simulink model "SmartGrid"  (R2023a)
settings: Solver=FixedStepDiscrete  StartTime=0.0  StopTime=20  FixedStep=1e-6  RelTol=1e-3
undefined symbols (not defined in the file or in its folder): Ion, Lithium
libraries: spsSeriesRLCBranchLib x7, spsCurrentMeasurementLib x3, spsPWMGeneratorDCDCLib x3, spsMosfetLib x2, spsVoltageMeasurementLib x2, spsBatteryLib x1, spsPVArrayLib x1, spsDiodeLib x1, spsIGBTDiodeLib x1, spspowerguiLib x1
settings Model: Creator=Dishan Dey  LastModifiedBy=Dishan Dey

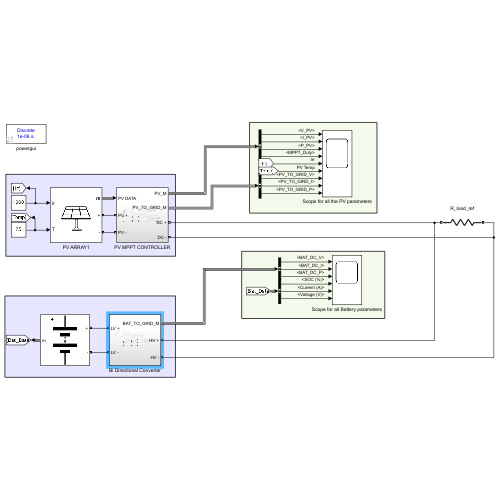
[thumbnail: Simulink's stored preview of the top-level diagram]
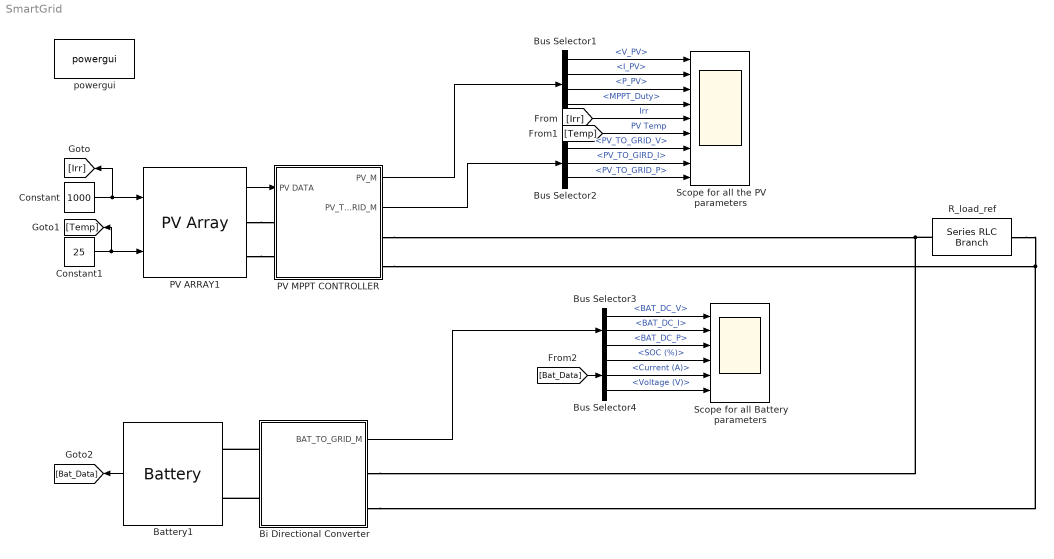
== system SmartGrid ==
  Battery1 : spsBatteryLib/Battery  BatType=Lithium-Ion  ShowTempParam=off  ThermalPreset=no  ShowAgeParam=off  NomV=48  NomQ=50  SOC=80  Batt_Tr=30  PresetModel=on  MaxQ=50  MinV=36  FullV=55.8714  Dis_rate=21.7391  R=0.0096  Normal_OP=45.2174  expZone="[51.8585      2.45652]"  current=[6.5 13 32.5]  Units=Time  Tci=20  NomT=20  T2=-30  MaxQ2=4.8  FullV2=7.1  Normal_OP2=5.655  expZone2="[6.58           1]"  Rca=0.6  ti=2000  Dp=0  Neq0=0  Tsim=1e6  Ta1=25  Qeol=5.4*0.9  Reol=0.013333*1.2  Char_age=[2.3478, 3]  Dis_age=[2.3478, 10]  N1=1500  N2=10500  N3=1000  N4=1400  Ta2=45  N5=950
  Bi Directional Converter : Subsystem
  Bus Selector1 : BusSelector  OutputSignals=V_PV,I_PV,P_PV,MPPT_Duty
  Bus Selector2 : BusSelector  OutputSignals=PV_TO_GRID_V,PV_TO_GIRD_I,PV_TO_GRID_P
  Bus Selector3 : BusSelector  OutputSignals=BAT_DC_V,BAT_DC_I,BAT_DC_P
  Bus Selector4 : BusSelector  OutputSignals=SOC (%),Current (A),Voltage (V)
  Constant : Constant  Value=1000  SampleTime=-1
  Constant1 : Constant  Value=25  SampleTime=-1
  PV ARRAY1 : spsPVArrayLib/PV Array  Npar=6  Nser=1  PlotType=array @ 25 deg.C & specified irradiances  S_vec="[ 1000  500  100 ]"  Temp_C_vec="[ 45 25  ]"  ModuleName=Canadian Solar Inc. CS6P-250P  PlotWhenSelected=off  Pm=249.83  Ncell=60  Voc=37.2  Isc=8.87  Vm=30.1  Im=8.3  beta_Voc_pc=-0.301  alpha_Isc_pc=0.038997  beta_Voc=-0.11197  alpha_Isc=0.003459  IL=8.8849  I0=3.0928e-11  nI=0.91537  Rsh=202.8148  Rs=0.34115  RobustModel=off  RobustCellTemperature=313.3991  BAL=on  Tc=1e-6  Tfilter=5e-5
  PV MPPT CONTROLLER : Subsystem
  R_load_ref : spsSeriesRLCBranchLib/Series RLC Branch  LConnTagsString=__new0  RConnTagsString=__new0  BranchType=R  Resistance=10  Inductance=1e-3  SetiL0=off  InitialCurrent=0  Capacitance=1e-6  Setx0=off  InitialVoltage=0  Measurements=None
  Scope for all Battery parameters : Scope  NumInputPorts=6
  Scope for all the PV parameters : Scope  NumInputPorts=9
  powergui : spspowerguiLib/powergui  Priority=1  SimulationMode=Discrete  SampleTime=1e-6  frequency=60  Iterations=50  frequencyindice=0  Pbase=100e6  ErrMax=1e-4  UnitsV=kV  UnitsW=MW  buscounter=0  FunctionMessages=off  echomessages=off  EnableUseOfTLC=off  CurrentSourceSwitches=off  DisableSnubberDevices=off  DisableRonSwitches=off  DisableVfSwitches=off  DisplayEquations=off  AutomaticDiscreteSolvers=off  SolverType=Tustin/Backward Euler (TBE)  Interpol=off  ExternalGateDelay=off  methode=off  Ts=100  x0status=blocks  SPID=on  SwTol=0  HookPort=off  NonlinearTolerance=1e-4  nMaxIteration=100  ContinueOnMaxIteration=off  RestoreLinks=warning  ResistiveCurrentMeasurement=off  Frange=[0:2:500]  Ylog=off  Xlog=on  ShowGrid=off  save=off  variable=ZData  structure=0  ZoomFFT=off  StartTime=0.0  cycles=1  DisplayStyle=1  fundamental=60  FreqAxis=off  MaxFrequency=1000  frequencyindicesteady=1  RmsSteady=1  display=off
  wires:
  PV ARRAY1/1 -> PV MPPT CONTROLLER/1(PV DATA)
  Constant/1 -> [Irr], PV ARRAY1/1
  Constant1/1 -> [Temp], PV ARRAY1/2
  PV MPPT CONTROLLER/1(PV_M) -> Bus Selector1/1
  Bus Selector1/1 -> Scope for all the PV parameters/1  "<V_PV>"
  Bus Selector1/2 -> Scope for all the PV parameters/2  "<I_PV>"
  Bus Selector1/3 -> Scope for all the PV parameters/3  "<P_PV>"
  PV MPPT CONTROLLER/2(PV_TO_GRID_M) -> Bus Selector2/1
  Bus Selector2/2 -> Scope for all the PV parameters/8  "<PV_TO_GIRD_I>"
  Bus Selector2/3 -> Scope for all the PV parameters/9  "<PV_TO_GRID_P>"
  Bi Directional Converter/1(BAT_TO_GRID_M) -> Bus Selector3/1
  Bus Selector3/1 -> Scope for all Battery parameters/1  "<BAT_DC_V>"
  Bus Selector3/2 -> Scope for all Battery parameters/2  "<BAT_DC_I>"
  Bus Selector3/3 -> Scope for all Battery parameters/3  "<BAT_DC_P>"
  Battery1/1 -> [Bat_Data]
  Bus Selector1/4 -> Scope for all the PV parameters/4  "<MPPT_Duty>"
  [Temp] -> Scope for all the PV parameters/6  "PV Temp"
  [Irr] -> Scope for all the PV parameters/5  "Irr"
  Bus Selector2/1 -> Scope for all the PV parameters/7  "<PV_TO_GRID_V>"
  Bus Selector4/2 -> Scope for all Battery parameters/5  "<Current (A)>"
  Bus Selector4/3 -> Scope for all Battery parameters/6  "<Voltage (V)>"
  Bus Selector4/1 -> Scope for all Battery parameters/4  "<SOC (%)>"
  [Bat_Data] -> Bus Selector4/1
  connections:
  PV ARRAY1/RConn1 -- PV MPPT CONTROLLER/LConn1
  PV ARRAY1/RConn2 -- PV MPPT CONTROLLER/LConn2
  PV MPPT CONTROLLER/RConn1 -- Bi Directional Converter/RConn1 -- R_load_ref/LConn1
  PV MPPT CONTROLLER/RConn2 -- Bi Directional Converter/RConn2 -- R_load_ref/RConn1
  Bi Directional Converter/LConn1 -- Battery1/LConn1
  Bi Directional Converter/LConn2 -- Battery1/LConn2

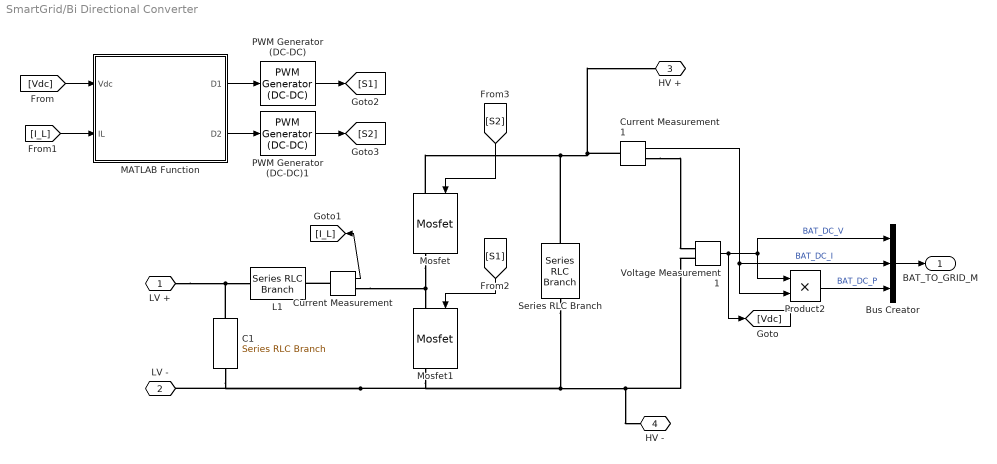
== system SmartGrid/Bi Directional Converter ==
  Bus Creator : BusCreator  Inputs=3
  C1 : spsSeriesRLCBranchLib/Series RLC Branch  LConnTagsString=__new0  RConnTagsString=__new0  BranchType=C  Resistance=1e-3  Inductance=1e-3  SetiL0=off  InitialCurrent=0  Capacitance=470e-06  Setx0=off  InitialVoltage=0  Measurements=None
  Current Measurement : spsCurrentMeasurementLib/Current Measurement  PhasorSimulation=off  OutputType=Complex  PSBequivalent=0
  Current Measurement1 : spsCurrentMeasurementLib/Current Measurement  PhasorSimulation=off  OutputType=Complex  PSBequivalent=0
  L1 : spsSeriesRLCBranchLib/Series RLC Branch  LConnTagsString=__new0  RConnTagsString=__new0  BranchType=L  Resistance=0.2e-3  Inductance=470e-6  SetiL0=off  InitialCurrent=0  Capacitance=1e-6  Setx0=off  InitialVoltage=0  Measurements=None
  MATLAB Function : MATLAB Function  TreatAsAtomicUnit=on
  Mosfet : spsMosfetLib/Mosfet  Ron=0.1  Lon=0  Rd=0.01  Vfd=0  IC=0  Rs=1e5  Cs=inf  Measurements=on
  Mosfet1 : spsMosfetLib/Mosfet  Ron=0.1  Lon=0  Rd=0.01  Vfd=0  IC=0  Rs=1e5  Cs=inf  Measurements=on
  PWM Generator (DC-DC) : spsPWMGeneratorDCDCLib/PWM Generator (DC-DC)  Fsw=10000  Ts=1e-06
  PWM Generator (DC-DC)1 : spsPWMGeneratorDCDCLib/PWM Generator (DC-DC)  Fsw=10000  Ts=1e-06
  Product2 : Product
  Series RLC Branch : spsSeriesRLCBranchLib/Series RLC Branch  LConnTagsString=__new0  RConnTagsString=__new0  BranchType=C  Resistance=1  Inductance=1e-3  SetiL0=off  InitialCurrent=0  Capacitance=1000e-06  Setx0=off  InitialVoltage=100  Measurements=None
  Voltage Measurement1 : spsVoltageMeasurementLib/Voltage Measurement  PhasorSimulation=off  OutputType=Complex  PSBequivalent=0
  LV + : PMIOPort  Side=Left
  LV - : PMIOPort  Port=2  Side=Left
  HV + : PMIOPort  Port=3  Side=Right
  HV - : PMIOPort  Port=4  Side=Right
  BAT_TO_GRID_M : Outport
  wires:
  [Vdc] -> MATLAB Function/1(Vdc)
  [I_L] -> MATLAB Function/2(IL)
  [S1] -> Mosfet1/1
  [S2] -> Mosfet/1
  Current Measurement1/1 -> Product2/2, Bus Creator/2  "BAT_DC_I"
  Product2/1 -> Bus Creator/3  "BAT_DC_P"
  Voltage Measurement1/1 -> [Vdc], Bus Creator/1, Product2/1  "BAT_DC_V"
  Bus Creator/1 -> BAT_TO_GRID_M/1
  MATLAB Function/1(D1) -> PWM Generator (DC-DC)/1
  MATLAB Function/2(D2) -> PWM Generator (DC-DC)1/1
  PWM Generator (DC-DC)/1 -> [S1]
  PWM Generator (DC-DC)1/1 -> [S2]
  Current Measurement/1 -> [I_L]
  connections:
  Mosfet/RConn1 -- Current Measurement/RConn1 -- Mosfet1/LConn1
  Mosfet/LConn1 -- Series RLC Branch/LConn1 -- Current Measurement1/LConn1 -- HV +/RConn1
  C1/LConn1 -- L1/RConn1 -- LV +/RConn1
  Voltage Measurement1/LConn2 -- Series RLC Branch/RConn1 -- Mosfet1/RConn1 -- C1/RConn1 -- LV -/RConn1 -- HV -/RConn1
  Current Measurement/LConn1 -- L1/LConn1
  Current Measurement1/RConn1 -- Voltage Measurement1/LConn1

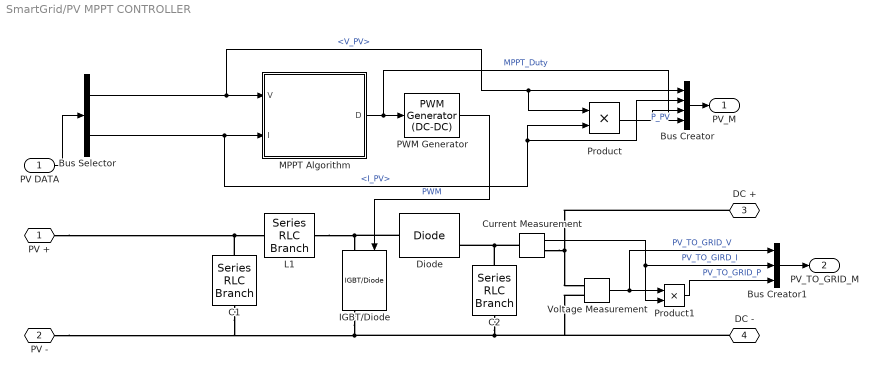
== system SmartGrid/PV MPPT CONTROLLER ==
  PV DATA : Inport
  Bus Creator : BusCreator  Inputs=4
  Bus Creator1 : BusCreator  Inputs=3
  Bus Selector : BusSelector  OutputSignals=V_PV,I_PV
  C1 : spsSeriesRLCBranchLib/Series RLC Branch  LConnTagsString=__new0  RConnTagsString=__new0  BranchType=C  Resistance=0.00100001  Inductance=1e-3  SetiL0=off  InitialCurrent=0  Capacitance=350e-6  Setx0=off  InitialVoltage=0  Measurements=None
  C2 : spsSeriesRLCBranchLib/Series RLC Branch  LConnTagsString=__new0  RConnTagsString=__new0  BranchType=C  Resistance=0.00000000001  Inductance=1e-3  SetiL0=off  InitialCurrent=0  Capacitance=470e-06  Setx0=off  InitialVoltage=100  Measurements=None
  Current Measurement : spsCurrentMeasurementLib/Current Measurement  PhasorSimulation=off  OutputType=Complex  PSBequivalent=0
  Diode : spsDiodeLib/Diode  Ron=0.001  Lon=0  Vf=0.8  IC=0  UseSnubber=0  Rs=500  Cs=250e-9  Measurements=on
  IGBT/Diode : spsIGBTDiodeLib/IGBT//Diode  Ron=1e-3  Rs=1e5  Cs=inf  Measurements=on
  L1 : spsSeriesRLCBranchLib/Series RLC Branch  LConnTagsString=__new0  RConnTagsString=__new0  BranchType=L  Resistance=1  Inductance=350e-06  SetiL0=off  InitialCurrent=0  Capacitance=1e-6  Setx0=off  InitialVoltage=0  Measurements=None
  MPPT Algorithm : MATLAB Function  TreatAsAtomicUnit=on
  PWM Generator : spsPWMGeneratorDCDCLib/PWM Generator (DC-DC)  Fsw=10000  Ts=1e-6
  Product : Product
  Product1 : Product
  Voltage Measurement : spsVoltageMeasurementLib/Voltage Measurement  PhasorSimulation=off  OutputType=Complex  PSBequivalent=0
  PV + : PMIOPort  Side=Left
  PV - : PMIOPort  Port=2  Side=Left
  DC + : PMIOPort  Port=3  Side=Right
  DC - : PMIOPort  Port=4  Side=Right
  PV_M : Outport
  PV_TO_GRID_M : Outport  Port=2
  wires:
  PV DATA/1 -> Bus Selector/1
  Product/1 -> Bus Creator/3  "P_PV"
  PWM Generator/1 -> IGBT/Diode/1  "PWM"
  Bus Creator/1 -> PV_M/1
  Bus Creator1/1 -> PV_TO_GRID_M/1
  Voltage Measurement/1 -> Bus Creator1/1, Product1/1  "PV_TO_GRID_V"
  Product1/1 -> Bus Creator1/3  "PV_TO_GRID_P"
  Current Measurement/1 -> Product1/2, Bus Creator1/2  "PV_TO_GIRD_I"
  Bus Selector/1 -> Product/1, Bus Creator/1, MPPT Algorithm/1(V)  "<V_PV>"
  Bus Selector/2 -> Bus Creator/2, Product/2, MPPT Algorithm/2(I)  "<I_PV>"
  MPPT Algorithm/1(D) -> Bus Creator/4, PWM Generator/1  "MPPT_Duty"
  connections:
  PV +/RConn1 -- C1/LConn1 -- L1/RConn1
  L1/LConn1 -- Diode/LConn1 -- IGBT/Diode/LConn1
  IGBT/Diode/RConn1 -- C2/RConn1 -- Voltage Measurement/LConn2 -- DC -/RConn1 -- C1/RConn1 -- PV -/RConn1
  Current Measurement/LConn1 -- C2/LConn1 -- Diode/RConn1
  Current Measurement/RConn1 -- DC +/RConn1 -- Voltage Measurement/LConn1

== matlab function SmartGrid/Bi Directional Converter/MATLAB Function ==
  settings: updateMethod=DISCRETE  sampleTime=1e-5
  data: Vdc input; D1 output; IL input; D2 output
function [D1, D2] = dc_bus_controller(Vdc, IL)

% ================================
% PARAMETERS
% ================================
Vref = 100;
Ts = 1e-5;

% Tuned gains (stable)
Kp_v = 0.4;
Ki_v = 30;
Kp_i = 0.03;

I_max = 30;

D_max = 0.9;
D_min = 0.05;

upper = 102;
lower = 98;

% ================================
% PERSISTENT
% ================================
persistent integral mode

if isempty(integral)
    integral = 0;
end

if isempty(mode)
    mode = 1; % start in BOOST
end

% ================================
% VOLTAGE CONTROL
% ================================
e = Vref - Vdc;

integral = integral + e * Ts;
integral = max(-20, min(20, integral)); % anti-windup

I_ref = Kp_v * e + Ki_v * integral;
I_ref = max(-I_max, min(I_max, I_ref));

% ================================
% MODE LOGIC (CLEAN)
% ================================
if Vdc > upper
    mode = 2; % BUCK
elseif Vdc < lower
    mode = 1; % BOOST
end

% ================================
% CURRENT CONTROL
% ================================
D = Kp_i * (I_ref - IL);

% Limit duty
D = max(D_min, min(D_max, abs(D)));

% ================================
% OUTPUT DUTIES (KEY PART)
% ================================
if mode == 1
    % BOOST MODE
    D1 = D;   % S1 active
    D2 = 0;   % S2 OFF
else
    % BUCK MODE
    D1 = 0;   % S1 OFF
    D2 = D;   % S2 active
end

end

== matlab function SmartGrid/PV MPPT CONTROLLER/MPPT Algorithm ==
  settings: updateMethod=DISCRETE  sampleTime=1e-4
  data: V input; I input; D output
function D = mppt_P_O(V, I)

persistent V_old P_old D_old

if isempty(V_old)
    V_old = V;
    P_old = V * I;
    D_old = 0.7;
end

deltaD = 0.002;
epsilon = 1e-6;

P = V * I;

dP = P - P_old;
dV = V - V_old;

if abs(dP) < epsilon
    D = D_old;
else
    if dP > 0
        if dV > 0
            D = D_old - deltaD;
        else
            D = D_old + deltaD;
        end
    else
        if dV > 0
            D = D_old + deltaD;
        else
            D = D_old - deltaD;
        end
    end
end

D = max(0.05, min(0.95, D));

V_old = V;
P_old = P;
D_old = D;

end
